simulink model "Seven_level_MCI_PMSM_Control"  (R2025a)
settings: Solver=VariableStepAuto  StartTime=0.0  StopTime=1  RelTol=1e-3
undefined symbols (not defined in the file or in its folder): Ion, Lithium
libraries: spsIGBTDiodeLib x36, spsCurrentMeasurementLib x15, spsBreakerLib x9, spsBatteryLib x9, spsVoltageMeasurementLib x6, spsRMSLib x3, slpidlib x1, spsGroundLib x1, spsPermanentMagnetSynchronousMachineLib x1, simulink x1, spsThreePhaseVIMeasurementLib x1, spspowerguiLib x1
(part 2 of 2)

== matlab function Seven_level_MCI_PMSM_Control/Controller/MATLAB Function2 ==
  data: L input; G1 output; G2 output; G3 output; G4 output; G5 output; G6 output; G7 output; G8 output; G9 output; G10 output; G11 output; G12 output
function [G1,G2,G3,G4,G5,G6,G7,G8,G9,G10,G11,G12] = CHB7_Gating(L)
%#codegen
% Input: L ∈ {-3,-2,-1,0,1,2,3}
% Output: 12 gate signals for 3 H-bridges (4 per bridge)

% Initialize all gate pulses to 0
G1=0; G2=0; G3=0; G4=0;
G5=0; G6=0; G7=0; G8=0;
G9=0; G10=0; G11=0; G12=0;

switch L
    case 3  % +3Vdc = +Vdc + +Vdc + +Vdc
        % All 3 H-bridges produce +Vdc
        [G1,G2,G3,G4]   = deal(1,1,0,0);
        [G5,G6,G7,G8]   = deal(1,1,0,0);
        [G9,G10,G11,G12]= deal(1,1,0,0);
        
    case 2  % +2Vdc = +Vdc + +Vdc + 0
        [G1,G2,G3,G4]   = deal(1,1,0,0);
        [G5,G6,G7,G8]   = deal(1,1,0,0);
        [G9,G10,G11,G12]= deal(0,1,1,0);
        
    case 1  % +Vdc = +Vdc + 0 + 0
        [G1,G2,G3,G4]   = deal(1,1,0,0);
        [G5,G6,G7,G8]   = deal(0,1,1,0);
        [G9,G10,G11,G12]= deal(0,1,1,0);
        
    case 0  % 0 = 0 + 0 + 0
        [G1,G2,G3,G4]   = deal(0,1,1,0);
        [G5,G6,G7,G8]   = deal(0,1,1,0);
        [G9,G10,G11,G12]= deal(0,1,1,0);
        
    case -1 % -Vdc = -Vdc + 0 + 0
        [G1,G2,G3,G4]   = deal(0,0,1,1);
        [G5,G6,G7,G8]   = deal(0,1,1,0);
        [G9,G10,G11,G12]= deal(0,1,1,0);
        
    case -2 % -2Vdc = -Vdc + -Vdc + 0
        [G1,G2,G3,G4]   = deal(0,0,1,1);
        [G5,G6,G7,G8]   = deal(0,0,1,1);
        [G9,G10,G11,G12]= deal(0,1,1,0);
        
    case -3 % -3Vdc = -Vdc + -Vdc + -Vdc
        [G1,G2,G3,G4]   = deal(0,0,1,1);
        [G5,G6,G7,G8]   = deal(0,0,1,1);
        [G9,G10,G11,G12]= deal(0,0,1,1);
end
end

== matlab function Seven_level_MCI_PMSM_Control/Controller/MATLAB Function3 ==
  data: L input; G1 output; G2 output; G3 output; G4 output; G5 output; G6 output; G7 output; G8 output; G9 output; G10 output; G11 output; G12 output
function [G1,G2,G3,G4,G5,G6,G7,G8,G9,G10,G11,G12] = CHB7_Gating(L)
%#codegen
% Input: L ∈ {-3,-2,-1,0,1,2,3}
% Output: 12 gate signals for 3 H-bridges (4 per bridge)

% Initialize all gate pulses to 0
G1=0; G2=0; G3=0; G4=0;
G5=0; G6=0; G7=0; G8=0;
G9=0; G10=0; G11=0; G12=0;

switch L
    case 3  % +3Vdc = +Vdc + +Vdc + +Vdc
        % All 3 H-bridges produce +Vdc
        [G1,G2,G3,G4]   = deal(1,1,0,0);
        [G5,G6,G7,G8]   = deal(1,1,0,0);
        [G9,G10,G11,G12]= deal(1,1,0,0);
        
    case 2  % +2Vdc = +Vdc + +Vdc + 0
        [G1,G2,G3,G4]   = deal(1,1,0,0);
        [G5,G6,G7,G8]   = deal(1,1,0,0);
        [G9,G10,G11,G12]= deal(0,1,1,0);
        
    case 1  % +Vdc = +Vdc + 0 + 0
        [G1,G2,G3,G4]   = deal(1,1,0,0);
        [G5,G6,G7,G8]   = deal(0,1,1,0);
        [G9,G10,G11,G12]= deal(0,1,1,0);
        
    case 0  % 0 = 0 + 0 + 0
        [G1,G2,G3,G4]   = deal(0,1,1,0);
        [G5,G6,G7,G8]   = deal(0,1,1,0);
        [G9,G10,G11,G12]= deal(0,1,1,0);
        
    case -1 % -Vdc = -Vdc + 0 + 0
        [G1,G2,G3,G4]   = deal(0,0,1,1);
        [G5,G6,G7,G8]   = deal(0,1,1,0);
        [G9,G10,G11,G12]= deal(0,1,1,0);
        
    case -2 % -2Vdc = -Vdc + -Vdc + 0
        [G1,G2,G3,G4]   = deal(0,0,1,1);
        [G5,G6,G7,G8]   = deal(0,0,1,1);
        [G9,G10,G11,G12]= deal(0,1,1,0);
        
    case -3 % -3Vdc = -Vdc + -Vdc + -Vdc
        [G1,G2,G3,G4]   = deal(0,0,1,1);
        [G5,G6,G7,G8]   = deal(0,0,1,1);
        [G9,G10,G11,G12]= deal(0,0,1,1);
end
end
